simulink model "Pedals_Susp_Sensors_ETR07"  (R2017b)
settings: Solver=FixedStepAuto  StartTime=0.0  StopTime=10.0  RelTol=1e-3
settings Model: Creator=cspt  LastModifiedBy=cspt
settings RTWCC: SystemTargetFile=irt.tlc  TemplateMakefile=irt_default_tmf  Description=INTECRIO Real-Time Target
settings STFCustomTargetCC: TargetLangStandard=C99 (ISO)  UtilityFuncGeneration=Shared location  SystemTargetFile=irt.tlc
settings GRTTargetCC: UtilityFuncGeneration=Shared location  ParMdlRefBuildCompliant=off  CompOptLevelCompliant=off  ConcurrentExecutionCompliant=off  CombineOutputUpdateFcns=off  MatFileLogging=off  CPPClassGenCompliant=off  GRTInterface=on  UseToolchainInfoCompliant=off  GenerateASAP2=on

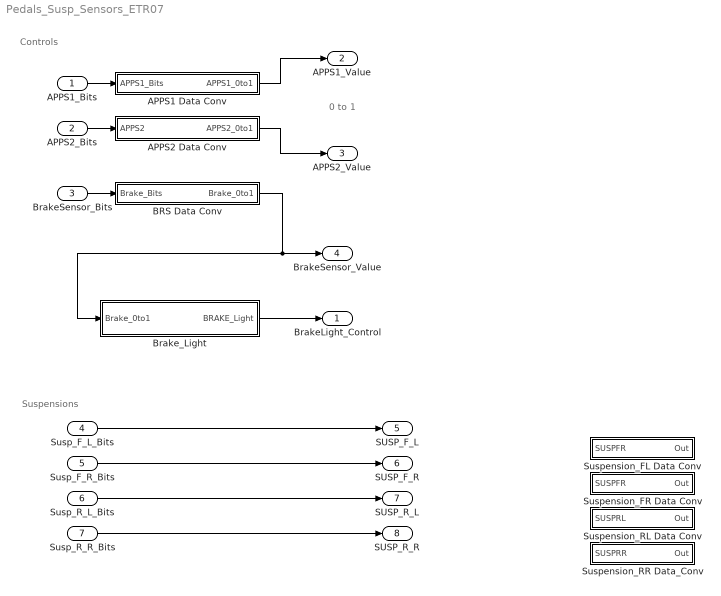
== system Pedals_Susp_Sensors_ETR07 ==
  note: 0 to 1
  note: Controls
  note: Suspensions
  APPS1_Bits : Inport
  APPS2_Bits : Inport  Port=2
  BrakeSensor_Bits : Inport  Port=3
  Susp_F_L_Bits : Inport  Port=4
  Susp_F_R_Bits : Inport  Port=5
  Susp_R_L_Bits : Inport  Port=6
  Susp_R_R_Bits : Inport  Port=7
  APPS1 Data Conv : Subsystem
  "APPS2 Data Conv " : Subsystem
  BRS Data Conv : Subsystem
  Brake_Light : Subsystem  TreatAsAtomicUnit=on
  Suspension_FL Data Conv : Subsystem
  Suspension_FR Data Conv : Subsystem
  Suspension_RL Data Conv : Subsystem
  Suspension_RR Data_Conv : Subsystem
  BrakeLight_Control : Outport
  APPS1_Value : Outport  Port=2
  APPS2_Value : Outport  Port=3
  BrakeSensor_Value : Outport  Port=4
  SUSP_F_L : Outport  Port=5
  SUSP_F_R : Outport  Port=6
  SUSP_R_L : Outport  Port=7
  SUSP_R_R : Outport  Port=8
  wires:
  APPS1 Data Conv/1(APPS1_0to1) -> APPS1_Value/1
  APPS1_Bits/1 -> APPS1 Data Conv/1(APPS1_Bits)
  BrakeSensor_Bits/1 -> BRS Data Conv/1(Brake_Bits)
  Brake_Light/1(BRAKE_Light) -> BrakeLight_Control/1
  BRS Data Conv/1(Brake_0to1) -> BrakeSensor_Value/1, Brake_Light/1(Brake_0to1)
  "APPS2 Data Conv "/1(APPS2_0to1) -> APPS2_Value/1
  APPS2_Bits/1 -> "APPS2 Data Conv "/1(APPS2)
  Susp_F_R_Bits/1 -> SUSP_F_R/1
  Susp_R_R_Bits/1 -> SUSP_R_R/1
  Susp_R_L_Bits/1 -> SUSP_R_L/1
  Susp_F_L_Bits/1 -> SUSP_F_L/1

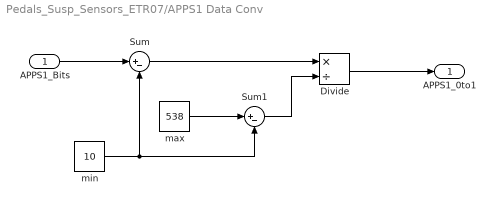
== system Pedals_Susp_Sensors_ETR07/APPS1 Data Conv ==
  APPS1_Bits : Inport
  Divide : Product  Inputs=*/
  Sum : Sum  Inputs=|+-
  Sum1 : Sum  Inputs=|+-
  max : Constant  Value=538
  min : Constant  Value=10
  APPS1_0to1 : Outport
  wires:
  APPS1_Bits/1 -> Sum/1
  min/1 -> Sum/2, Sum1/2
  max/1 -> Sum1/1
  Sum/1 -> Divide/1
  Sum1/1 -> Divide/2
  Divide/1 -> APPS1_0to1/1

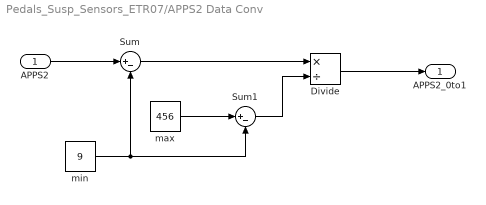
== system Pedals_Susp_Sensors_ETR07/APPS2 Data Conv  ==
  APPS2 : Inport
  Divide : Product  Inputs=*/
  Sum : Sum  Inputs=|+-
  Sum1 : Sum  Inputs=|+-
  max : Constant  Value=456
  min : Constant  Value=9
  APPS2_0to1 : Outport
  wires:
  APPS2/1 -> Sum/1
  min/1 -> Sum/2, Sum1/2
  max/1 -> Sum1/1
  Sum/1 -> Divide/1
  Sum1/1 -> Divide/2
  Divide/1 -> APPS2_0to1/1

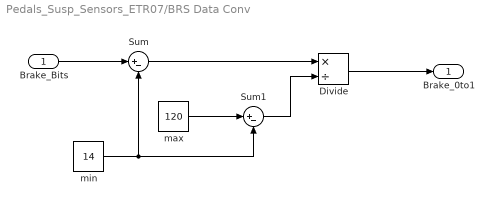
== system Pedals_Susp_Sensors_ETR07/BRS Data Conv ==
  Brake_Bits : Inport
  Divide : Product  Inputs=*/
  Sum : Sum  Inputs=|+-
  Sum1 : Sum  Inputs=|+-
  max : Constant  Value=120
  min : Constant  Value=14
  Brake_0to1 : Outport
  wires:
  Brake_Bits/1 -> Sum/1
  min/1 -> Sum/2, Sum1/2
  max/1 -> Sum1/1
  Sum/1 -> Divide/1
  Sum1/1 -> Divide/2
  Divide/1 -> Brake_0to1/1

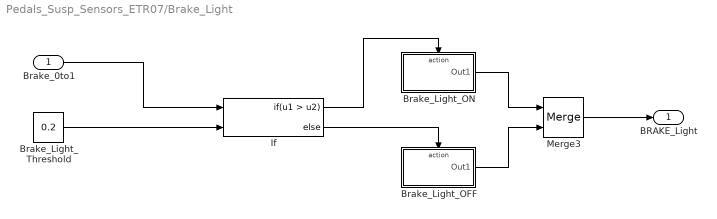
== system Pedals_Susp_Sensors_ETR07/Brake_Light ==
  Brake_0to1 : Inport
  Brake_Light_OFF : Subsystem  TreatAsAtomicUnit=on
  Brake_Light_ON : Subsystem  TreatAsAtomicUnit=on
  Brake_Light_Threshold : Constant  Value=0.2
  If : If  NumInputs=2  IfExpression=u1 > u2
  Merge3 : Merge
  BRAKE_Light : Outport
  wires:
  Brake_Light_Threshold/1 -> If/2
  If/1 -> Brake_Light_ON/Action
  If/2 -> Brake_Light_OFF/Action
  Brake_Light_ON/1(Out1) -> Merge3/1
  Brake_Light_OFF/1(Out1) -> Merge3/2
  Merge3/1 -> BRAKE_Light/1
  Brake_0to1/1 -> If/1

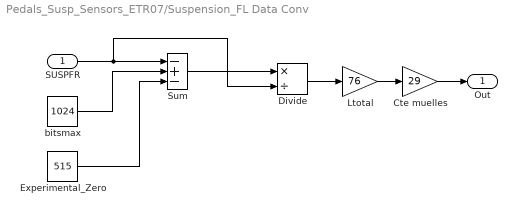
== system Pedals_Susp_Sensors_ETR07/Suspension_FL Data Conv ==
  SUSPFR : Inport
  Cte muelles : Gain  Gain=29
  Divide : Product  Inputs=*/
  Experimental_Zero : Constant  Value=515
  Ltotal : Gain  Gain=76
  Sum : Sum  Inputs=-+-
  "bitsmax " : Constant  Value=1024
  Out : Outport
  wires:
  Sum/1 -> Divide/1
  Divide/1 -> Ltotal/1
  Cte muelles/1 -> Out/1
  Ltotal/1 -> Cte muelles/1
  SUSPFR/1 -> Divide/2, Sum/1
  "bitsmax "/1 -> Sum/2
  Experimental_Zero/1 -> Sum/3

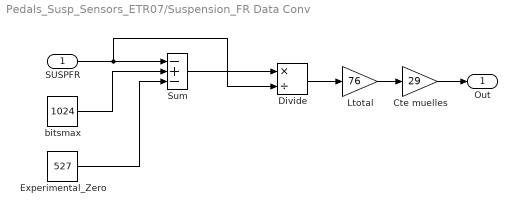
== system Pedals_Susp_Sensors_ETR07/Suspension_FR Data Conv ==
  SUSPFR : Inport
  Cte muelles : Gain  Gain=29
  Divide : Product  Inputs=*/
  Experimental_Zero : Constant  Value=527
  Ltotal : Gain  Gain=76
  Sum : Sum  Inputs=-+-
  "bitsmax " : Constant  Value=1024
  Out : Outport
  wires:
  Sum/1 -> Divide/1
  Divide/1 -> Ltotal/1
  Cte muelles/1 -> Out/1
  Ltotal/1 -> Cte muelles/1
  SUSPFR/1 -> Divide/2, Sum/1
  "bitsmax "/1 -> Sum/2
  Experimental_Zero/1 -> Sum/3

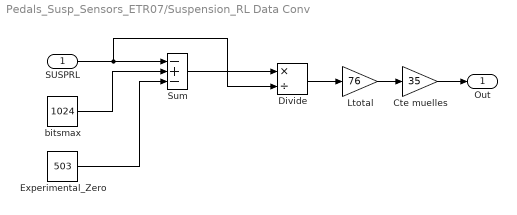
== system Pedals_Susp_Sensors_ETR07/Suspension_RL Data Conv ==
  SUSPRL : Inport
  Cte muelles : Gain  Gain=35
  Divide : Product  Inputs=*/
  Experimental_Zero : Constant  Value=503
  Ltotal : Gain  Gain=76
  Sum : Sum  Inputs=-+-
  "bitsmax " : Constant  Value=1024
  Out : Outport
  wires:
  Sum/1 -> Divide/1
  Divide/1 -> Ltotal/1
  Cte muelles/1 -> Out/1
  Ltotal/1 -> Cte muelles/1
  SUSPRL/1 -> Divide/2, Sum/1
  "bitsmax "/1 -> Sum/2
  Experimental_Zero/1 -> Sum/3

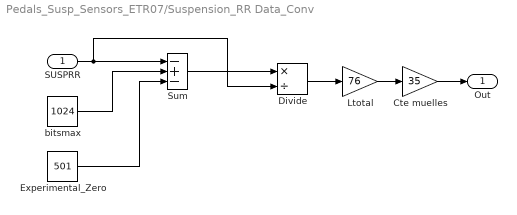
== system Pedals_Susp_Sensors_ETR07/Suspension_RR Data_Conv ==
  SUSPRR : Inport
  Cte muelles : Gain  Gain=35
  Divide : Product  Inputs=*/
  Experimental_Zero : Constant  Value=501
  Ltotal : Gain  Gain=76
  Sum : Sum  Inputs=-+-
  "bitsmax " : Constant  Value=1024
  Out : Outport
  wires:
  Sum/1 -> Divide/1
  Divide/1 -> Ltotal/1
  Cte muelles/1 -> Out/1
  Ltotal/1 -> Cte muelles/1
  SUSPRR/1 -> Sum/1, Divide/2
  "bitsmax "/1 -> Sum/2
  Experimental_Zero/1 -> Sum/3

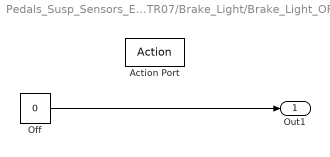
== system Pedals_Susp_Sensors_ETR07/Brake_Light/Brake_Light_OFF ==
  Action Port : ActionPort  ActionType=else
  Off : Constant  Value=0
  Out1 : Outport
  wires:
  Off/1 -> Out1/1

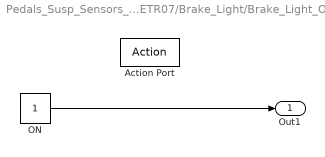
== system Pedals_Susp_Sensors_ETR07/Brake_Light/Brake_Light_ON ==
  Action Port : ActionPort  ActionType=then
  ON : Constant
  Out1 : Outport
  wires:
  ON/1 -> Out1/1
